simulink model "Deadbeat"  (R2017b)
settings: Solver=VariableStepAuto  StartTime=0.0  StopTime=50  RelTol=1e-3
settings Model: Creator=shayan  LastModifiedBy=shayan

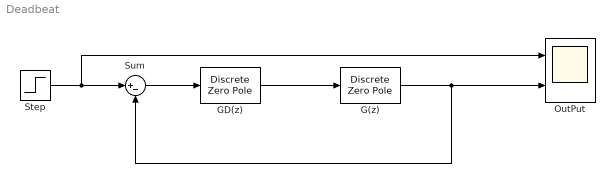
== system Deadbeat ==
  "G(z) " : DiscreteZeroPole  Zeros=[-2.8306 -0.1967 ]  Poles=[1 0.7788 0.3972]  Gain=-6.1431e-04  SampleTime=10
  "GD(z) " : DiscreteZeroPole  Zeros=[0.7788 0.3972]  Poles=[-0.7389 -0.1967]  Gain=0.261/(-6.1431*10^-4)  SampleTime=10
  "OutPut " : Scope  NumInputPorts=2
  Step : Step  SampleTime=0
  Sum : Sum  Inputs=|+-
  wires:
  "GD(z) "/1 -> "G(z) "/1
  Step/1 -> "OutPut "/1, Sum/1
  Sum/1 -> "GD(z) "/1
  "G(z) "/1 -> "OutPut "/2, Sum/2
